simulink model "indy7_dualArm"  (R2024b)
settings: Solver=FixedStepAuto  StartTime=0.0  StopTime=10  FixedStep=0.001  RelTol=1e-3
model workspace (MAT data in the model file):
  joint_friction = [80 80 20 10 10 5]
  lambda_l_list = [0 -1.17357539658 0.993815552956 -2.091 0 0 -0.111945470246 0.0246912114191 0.243747835972 1.20917417944 1.20917417944 -1.20905770917 ... (42 elements, 6x7)]
  lambda_r_list = [0 1.17618914658 0.992300581915 2.091 0 0 -0.111945470246 0.0246912114191 0.243747835972 1.20917417944 1.20917417944 -1.20905770917 ... (42 elements, 6x7)]
  lambda_rl_list = [2.58853268681e-20 -2.25514051877e-16 -0.06 -1.83339582048e-16 -4.06575814682e-20 0 0.0911029490978 -0.02862210596 -0.174516399919 1.20917417944 1.20905770917 -1.20917417944 ... (78 elements, 6x13)]
  q_init_l : Simulink.Parameter (value not decoded)
  q_init_l1 : Simulink.Parameter (value not decoded)
  q_init_l2 : Simulink.Parameter (value not decoded)
  q_init_l3 : Simulink.Parameter (value not decoded)
  q_init_l4 : Simulink.Parameter (value not decoded)
  q_init_l5 : Simulink.Parameter (value not decoded)
  q_init_l6 : Simulink.Parameter (value not decoded)
  q_init_r : Simulink.Parameter (value not decoded)
  q_init_r1 : Simulink.Parameter (value not decoded)
  q_init_r2 : Simulink.Parameter (value not decoded)
  q_init_r3 : Simulink.Parameter (value not decoded)
  q_init_r4 : Simulink.Parameter (value not decoded)
  q_init_r5 : Simulink.Parameter (value not decoded)
  q_init_r6 : Simulink.Parameter (value not decoded)
  robot : robotics.RigidBodyTree (value not decoded)
values from neighbouring files (symbols this model uses):
  lambda_lr_list = [lambda_lr_list,-lambda_rl_list(:,i)]    [getDualArmLambdaList.m]    (also in untitled3.m)
  m = models{k}    [code_generation.m]
  N = length(q)    [FKLocalPOE.m]
symbols that are objects in the model workspace (value not decoded): q_init_l, q_init_l1, q_init_r
undefined symbols (not defined in the file or in its folder): Blist_tcp, DiscIntNeverNeededParam, dt, exp6, M_tcp, q_init, q_max, q_min, qdot_max, qdot_min, SW_a, SW_b0, X, Y, Z
libraries: sm_lib x148, nesl_utility x45, robotmaniplib x9, robotcorelib x5, simulink x4, matrix_library x2
(part 4 of 5)

== system indy7_dualArm/DualArm/Right/r_3 ==
  Inertia : sm_lib/Body Elements/Inertia  InertiaType=Custom  Mass=2.99134127  MassUnits=kg  CenterOfMass=[0, 0, 0]  CenterOfMassUnits=m  MomentsOfInertia=[0.03424593, 0.03406024, 0.00450477]  MomentsOfInertiaUnits=kg*m^2  ProductsOfInertia=[0.00186009, 7.24e-06, 1.49e-06]  ProductsOfInertiaUnits=kg*m^2  GraphicType=None  MarkerShape=Inertia  MarkerSize=20  GraphicVisPropType=SimpleVisualProperties  GraphicDiffuseColor=[0.5 0.5 0.5]  GraphicOpacity=1  GraphicSpecularColor=[0.5 0.5 0.5 1.0]  GraphicAmbientColor=[0.15 0.15 0.15 1.0]  GraphicEmissiveColor=[0.0 0.0 0.0 1.0]  GraphicShininess=75
  InertiaOriginTransform : sm_lib/Frames and Transforms/Rigid Transform  RotationMethod=RotationSequence  FollAlignAxisA=+X  BaseAlignAxisA=+Y  FollAlignAxisB=+Y  BaseAlignAxisB=+Z  RotationStandardAxis=+Z  RotationAngle=0  RotationAngleUnits=deg  RotationArbitraryAxis=[0 0 1]  RotationSequenceAxes=BaseAxes  RotationSequence=XYZ  RotationSequenceAngles=[0, 0, 0]  RotationSequenceAnglesUnits=rad  RotationMatrix=[1 0 0;0 1 0;0 0 1]  Quaternion=[1 0 0 0]  TranslationMethod=Cartesian  TranslationCartesianOffset=[0, 0, 0]  TranslationCartesianOffsetUnits=m  TranslationStandardAxis=+Z  TranslationStandardOffset=0  TranslationStandardOffsetUnits=m  TranslationROffset=0  TranslationROffsetUnits=m  TranslationThetaOffset=0  TranslationThetaOffsetUnits=deg  TranslationZOffset=0  TranslationZOffsetUnits=m
  ReferenceFrame : sm_lib/Frames and Transforms/Reference Frame
  Visual : sm_lib/Body Elements/File Solid  ExtGeomFileName=meshes/visual/Indy7_3.stl  UnitType=Custom  ExtGeomFileUnits=m  StepReaderType=HEX  ExportConvexHullGeometry=off  InertiaType=Custom  BasedOnType=DensityFromFile  Density=1000  DensityUnits=kg/m^3  Mass=0  MassUnits=kg  CenterOfMass=[0, 0, 0]  CenterOfMassUnits=m  MomentsOfInertia=[0, 0, 0]  MomentsOfInertiaUnits=kg*m^2  ProductsOfInertia=[0, 0, 0]  ProductsOfInertiaUnits=kg*m^2  GraphicType=FromGeometry  MarkerShape=Sphere  MarkerSize=10  GraphicVisPropType=SimpleVisualProperties  GraphicDiffuseColor=[1,1,1]  GraphicOpacity=1  GraphicSpecularColor=[0.5 0.5 0.5 1.0]  GraphicAmbientColor=[0.15 0.15 0.15 1.0]  GraphicEmissiveColor=[0.0 0.0 0.0 1.0]  GraphicShininess=75  DoExposeReferenceFrame=on  SerializedFrames=<Frames/>
  VisualOriginTransform : sm_lib/Frames and Transforms/Rigid Transform  RotationMethod=RotationSequence  FollAlignAxisA=+X  BaseAlignAxisA=+Y  FollAlignAxisB=+Y  BaseAlignAxisB=+Z  RotationStandardAxis=+Z  RotationAngle=0  RotationAngleUnits=deg  RotationArbitraryAxis=[0 0 1]  RotationSequenceAxes=BaseAxes  RotationSequence=XYZ  RotationSequenceAngles=[0, 0, 0]  RotationSequenceAnglesUnits=rad  RotationMatrix=[1 0 0;0 1 0;0 0 1]  Quaternion=[1 0 0 0]  TranslationMethod=Cartesian  TranslationCartesianOffset=[0, 0, 0]  TranslationCartesianOffsetUnits=m  TranslationStandardAxis=+Z  TranslationStandardOffset=0  TranslationStandardOffsetUnits=m  TranslationROffset=0  TranslationROffsetUnits=m  TranslationThetaOffset=0  TranslationThetaOffsetUnits=deg  TranslationZOffset=0  TranslationZOffsetUnits=m
  r_joint_2_AxisInvTransform : sm_lib/Frames and Transforms/Rigid Transform  RotationMethod=ArbitraryAxis  FollAlignAxisA=+X  BaseAlignAxisA=+Y  FollAlignAxisB=+Y  BaseAlignAxisB=+Z  RotationStandardAxis=+Z  RotationAngle=0  RotationAngleUnits=rad  RotationArbitraryAxis=[1, 0, 0]  RotationSequenceAxes=FollowerAxes  RotationSequence=XYX  RotationSequenceAngles=[0 0 0]  RotationSequenceAnglesUnits=deg  RotationMatrix=[1 0 0;0 1 0;0 0 1]  Quaternion=[1 0 0 0]  TranslationMethod=Cartesian  TranslationCartesianOffset=[0, 0, 0]  TranslationCartesianOffsetUnits=m  TranslationStandardAxis=+Z  TranslationStandardOffset=0  TranslationStandardOffsetUnits=m  TranslationROffset=0  TranslationROffsetUnits=m  TranslationThetaOffset=0  TranslationThetaOffsetUnits=deg  TranslationZOffset=0  TranslationZOffsetUnits=m
  r_joint_3_AxisTransform : sm_lib/Frames and Transforms/Rigid Transform  RotationMethod=ArbitraryAxis  FollAlignAxisA=+X  BaseAlignAxisA=+Y  FollAlignAxisB=+Y  BaseAlignAxisB=+Z  RotationStandardAxis=+Z  RotationAngle=0  RotationAngleUnits=rad  RotationArbitraryAxis=[1, 0, 0]  RotationSequenceAxes=FollowerAxes  RotationSequence=XYX  RotationSequenceAngles=[0 0 0]  RotationSequenceAnglesUnits=deg  RotationMatrix=[1 0 0;0 1 0;0 0 1]  Quaternion=[1 0 0 0]  TranslationMethod=Cartesian  TranslationCartesianOffset=[0, 0, 0]  TranslationCartesianOffsetUnits=m  TranslationStandardAxis=+Z  TranslationStandardOffset=0  TranslationStandardOffsetUnits=m  TranslationROffset=0  TranslationROffsetUnits=m  TranslationThetaOffset=0  TranslationThetaOffsetUnits=deg  TranslationZOffset=0  TranslationZOffsetUnits=m
  r_joint_3_OriginTransform : sm_lib/Frames and Transforms/Rigid Transform  RotationMethod=RotationSequence  FollAlignAxisA=+X  BaseAlignAxisA=+Y  FollAlignAxisB=+Y  BaseAlignAxisB=+Z  RotationStandardAxis=+Z  RotationAngle=0  RotationAngleUnits=deg  RotationArbitraryAxis=[0 0 1]  RotationSequenceAxes=BaseAxes  RotationSequence=XYZ  RotationSequenceAngles=[-1.5707, 0, 1.5707]  RotationSequenceAnglesUnits=rad  RotationMatrix=[1 0 0;0 1 0;0 0 1]  Quaternion=[1 0 0 0]  TranslationMethod=Cartesian  TranslationCartesianOffset=[-0.267, 0, -0.075]  TranslationCartesianOffsetUnits=m  TranslationStandardAxis=+Z  TranslationStandardOffset=0  TranslationStandardOffsetUnits=m  TranslationROffset=0  TranslationROffsetUnits=m  TranslationThetaOffset=0  TranslationThetaOffsetUnits=deg  TranslationZOffset=0  TranslationZOffsetUnits=m
  F : PMIOPort  Side=Left
  F1 : PMIOPort  Port=2  Side=Right
  connections:
  Inertia/RConn1 -- InertiaOriginTransform/RConn1
  r_joint_2_AxisInvTransform/LConn1 -- r_joint_3_OriginTransform/LConn1 -- InertiaOriginTransform/LConn1 -- ReferenceFrame/RConn1 -- VisualOriginTransform/LConn1
  Visual/RConn1 -- VisualOriginTransform/RConn1
  r_joint_2_AxisInvTransform/RConn1 -- F/RConn1
  r_joint_3_AxisTransform/RConn1 -- F1/RConn1
  r_joint_3_AxisTransform/LConn1 -- r_joint_3_OriginTransform/RConn1

== system indy7_dualArm/DualArm/Right/r_4 ==
  Inertia : sm_lib/Body Elements/Inertia  InertiaType=Custom  Mass=2.12317035  MassUnits=kg  CenterOfMass=[0, 0, 0]  CenterOfMassUnits=m  MomentsOfInertia=[0.00670405, 0.00279246, 0.00619341]  MomentsOfInertiaUnits=kg*m^2  ProductsOfInertia=[-0.00127967, 1.5e-06, 3.75e-06]  ProductsOfInertiaUnits=kg*m^2  GraphicType=None  MarkerShape=Inertia  MarkerSize=20  GraphicVisPropType=SimpleVisualProperties  GraphicDiffuseColor=[0.5 0.5 0.5]  GraphicOpacity=1  GraphicSpecularColor=[0.5 0.5 0.5 1.0]  GraphicAmbientColor=[0.15 0.15 0.15 1.0]  GraphicEmissiveColor=[0.0 0.0 0.0 1.0]  GraphicShininess=75
  InertiaOriginTransform : sm_lib/Frames and Transforms/Rigid Transform  RotationMethod=RotationSequence  FollAlignAxisA=+X  BaseAlignAxisA=+Y  FollAlignAxisB=+Y  BaseAlignAxisB=+Z  RotationStandardAxis=+Z  RotationAngle=0  RotationAngleUnits=deg  RotationArbitraryAxis=[0 0 1]  RotationSequenceAxes=BaseAxes  RotationSequence=XYZ  RotationSequenceAngles=[0, 0, 0]  RotationSequenceAnglesUnits=rad  RotationMatrix=[1 0 0;0 1 0;0 0 1]  Quaternion=[1 0 0 0]  TranslationMethod=Cartesian  TranslationCartesianOffset=[0, 0, 0]  TranslationCartesianOffsetUnits=m  TranslationStandardAxis=+Z  TranslationStandardOffset=0  TranslationStandardOffsetUnits=m  TranslationROffset=0  TranslationROffsetUnits=m  TranslationThetaOffset=0  TranslationThetaOffsetUnits=deg  TranslationZOffset=0  TranslationZOffsetUnits=m
  ReferenceFrame : sm_lib/Frames and Transforms/Reference Frame
  Visual : sm_lib/Body Elements/File Solid  ExtGeomFileName=meshes/visual/Indy7_4.stl  UnitType=Custom  ExtGeomFileUnits=m  StepReaderType=HEX  ExportConvexHullGeometry=off  InertiaType=Custom  BasedOnType=DensityFromFile  Density=1000  DensityUnits=kg/m^3  Mass=0  MassUnits=kg  CenterOfMass=[0, 0, 0]  CenterOfMassUnits=m  MomentsOfInertia=[0, 0, 0]  MomentsOfInertiaUnits=kg*m^2  ProductsOfInertia=[0, 0, 0]  ProductsOfInertiaUnits=kg*m^2  GraphicType=FromGeometry  MarkerShape=Sphere  MarkerSize=10  GraphicVisPropType=SimpleVisualProperties  GraphicDiffuseColor=[1,1,1]  GraphicOpacity=1  GraphicSpecularColor=[0.5 0.5 0.5 1.0]  GraphicAmbientColor=[0.15 0.15 0.15 1.0]  GraphicEmissiveColor=[0.0 0.0 0.0 1.0]  GraphicShininess=75  DoExposeReferenceFrame=on  SerializedFrames=<Frames/>
  VisualOriginTransform : sm_lib/Frames and Transforms/Rigid Transform  RotationMethod=RotationSequence  FollAlignAxisA=+X  BaseAlignAxisA=+Y  FollAlignAxisB=+Y  BaseAlignAxisB=+Z  RotationStandardAxis=+Z  RotationAngle=0  RotationAngleUnits=deg  RotationArbitraryAxis=[0 0 1]  RotationSequenceAxes=BaseAxes  RotationSequence=XYZ  RotationSequenceAngles=[0, 0, 0]  RotationSequenceAnglesUnits=rad  RotationMatrix=[1 0 0;0 1 0;0 0 1]  Quaternion=[1 0 0 0]  TranslationMethod=Cartesian  TranslationCartesianOffset=[0, 0, 0]  TranslationCartesianOffsetUnits=m  TranslationStandardAxis=+Z  TranslationStandardOffset=0  TranslationStandardOffsetUnits=m  TranslationROffset=0  TranslationROffsetUnits=m  TranslationThetaOffset=0  TranslationThetaOffsetUnits=deg  TranslationZOffset=0  TranslationZOffsetUnits=m
  r_joint_3_AxisInvTransform : sm_lib/Frames and Transforms/Rigid Transform  RotationMethod=ArbitraryAxis  FollAlignAxisA=+X  BaseAlignAxisA=+Y  FollAlignAxisB=+Y  BaseAlignAxisB=+Z  RotationStandardAxis=+Z  RotationAngle=0  RotationAngleUnits=rad  RotationArbitraryAxis=[1, 0, 0]  RotationSequenceAxes=FollowerAxes  RotationSequence=XYX  RotationSequenceAngles=[0 0 0]  RotationSequenceAnglesUnits=deg  RotationMatrix=[1 0 0;0 1 0;0 0 1]  Quaternion=[1 0 0 0]  TranslationMethod=Cartesian  TranslationCartesianOffset=[0, 0, 0]  TranslationCartesianOffsetUnits=m  TranslationStandardAxis=+Z  TranslationStandardOffset=0  TranslationStandardOffsetUnits=m  TranslationROffset=0  TranslationROffsetUnits=m  TranslationThetaOffset=0  TranslationThetaOffsetUnits=deg  TranslationZOffset=0  TranslationZOffsetUnits=m
  r_joint_4_AxisTransform : sm_lib/Frames and Transforms/Rigid Transform  RotationMethod=ArbitraryAxis  FollAlignAxisA=+X  BaseAlignAxisA=+Y  FollAlignAxisB=+Y  BaseAlignAxisB=+Z  RotationStandardAxis=+Z  RotationAngle=0  RotationAngleUnits=rad  RotationArbitraryAxis=[1, 0, 0]  RotationSequenceAxes=FollowerAxes  RotationSequence=XYX  RotationSequenceAngles=[0 0 0]  RotationSequenceAnglesUnits=deg  RotationMatrix=[1 0 0;0 1 0;0 0 1]  Quaternion=[1 0 0 0]  TranslationMethod=Cartesian  TranslationCartesianOffset=[0, 0, 0]  TranslationCartesianOffsetUnits=m  TranslationStandardAxis=+Z  TranslationStandardOffset=0  TranslationStandardOffsetUnits=m  TranslationROffset=0  TranslationROffsetUnits=m  TranslationThetaOffset=0  TranslationThetaOffsetUnits=deg  TranslationZOffset=0  TranslationZOffsetUnits=m
  r_joint_4_OriginTransform : sm_lib/Frames and Transforms/Rigid Transform  RotationMethod=RotationSequence  FollAlignAxisA=+X  BaseAlignAxisA=+Y  FollAlignAxisB=+Y  BaseAlignAxisB=+Z  RotationStandardAxis=+Z  RotationAngle=0  RotationAngleUnits=deg  RotationArbitraryAxis=[0 0 1]  RotationSequenceAxes=BaseAxes  RotationSequence=XYZ  RotationSequenceAngles=[1.5707, 1.5707, 0]  RotationSequenceAnglesUnits=rad  RotationMatrix=[1 0 0;0 1 0;0 0 1]  Quaternion=[1 0 0 0]  TranslationMethod=Cartesian  TranslationCartesianOffset=[0, -0.114, 0.083]  TranslationCartesianOffsetUnits=m  TranslationStandardAxis=+Z  TranslationStandardOffset=0  TranslationStandardOffsetUnits=m  TranslationROffset=0  TranslationROffsetUnits=m  TranslationThetaOffset=0  TranslationThetaOffsetUnits=deg  TranslationZOffset=0  TranslationZOffsetUnits=m
  F : PMIOPort  Side=Left
  F1 : PMIOPort  Port=2  Side=Right
  connections:
  Inertia/RConn1 -- InertiaOriginTransform/RConn1
  r_joint_3_AxisInvTransform/LConn1 -- r_joint_4_OriginTransform/LConn1 -- InertiaOriginTransform/LConn1 -- ReferenceFrame/RConn1 -- VisualOriginTransform/LConn1
  Visual/RConn1 -- VisualOriginTransform/RConn1
  r_joint_3_AxisInvTransform/RConn1 -- F/RConn1
  r_joint_4_AxisTransform/RConn1 -- F1/RConn1
  r_joint_4_AxisTransform/LConn1 -- r_joint_4_OriginTransform/RConn1

== system indy7_dualArm/DualArm/Right/r_5 ==
  Inertia : sm_lib/Body Elements/Inertia  InertiaType=Custom  Mass=2.28865091  MassUnits=kg  CenterOfMass=[0, 0, 0]  CenterOfMassUnits=m  MomentsOfInertia=[0.00994891, 0.00978189, 0.00271492]  MomentsOfInertiaUnits=kg*m^2  ProductsOfInertia=[-0.00093546, 3.21e-06, 1.4e-07]  ProductsOfInertiaUnits=kg*m^2  GraphicType=None  MarkerShape=Inertia  MarkerSize=20  GraphicVisPropType=SimpleVisualProperties  GraphicDiffuseColor=[0.5 0.5 0.5]  GraphicOpacity=1  GraphicSpecularColor=[0.5 0.5 0.5 1.0]  GraphicAmbientColor=[0.15 0.15 0.15 1.0]  GraphicEmissiveColor=[0.0 0.0 0.0 1.0]  GraphicShininess=75
  InertiaOriginTransform : sm_lib/Frames and Transforms/Rigid Transform  RotationMethod=RotationSequence  FollAlignAxisA=+X  BaseAlignAxisA=+Y  FollAlignAxisB=+Y  BaseAlignAxisB=+Z  RotationStandardAxis=+Z  RotationAngle=0  RotationAngleUnits=deg  RotationArbitraryAxis=[0 0 1]  RotationSequenceAxes=BaseAxes  RotationSequence=XYZ  RotationSequenceAngles=[0, 0, 0]  RotationSequenceAnglesUnits=rad  RotationMatrix=[1 0 0;0 1 0;0 0 1]  Quaternion=[1 0 0 0]  TranslationMethod=Cartesian  TranslationCartesianOffset=[0, 0, 0]  TranslationCartesianOffsetUnits=m  TranslationStandardAxis=+Z  TranslationStandardOffset=0  TranslationStandardOffsetUnits=m  TranslationROffset=0  TranslationROffsetUnits=m  TranslationThetaOffset=0  TranslationThetaOffsetUnits=deg  TranslationZOffset=0  TranslationZOffsetUnits=m
  ReferenceFrame : sm_lib/Frames and Transforms/Reference Frame
  Visual : sm_lib/Body Elements/File Solid  ExtGeomFileName=meshes/visual/Indy7_5.stl  UnitType=Custom  ExtGeomFileUnits=m  StepReaderType=HEX  ExportConvexHullGeometry=off  InertiaType=Custom  BasedOnType=DensityFromFile  Density=1000  DensityUnits=kg/m^3  Mass=0  MassUnits=kg  CenterOfMass=[0, 0, 0]  CenterOfMassUnits=m  MomentsOfInertia=[0, 0, 0]  MomentsOfInertiaUnits=kg*m^2  ProductsOfInertia=[0, 0, 0]  ProductsOfInertiaUnits=kg*m^2  GraphicType=FromGeometry  MarkerShape=Sphere  MarkerSize=10  GraphicVisPropType=SimpleVisualProperties  GraphicDiffuseColor=[1,1,1]  GraphicOpacity=1  GraphicSpecularColor=[0.5 0.5 0.5 1.0]  GraphicAmbientColor=[0.15 0.15 0.15 1.0]  GraphicEmissiveColor=[0.0 0.0 0.0 1.0]  GraphicShininess=75  DoExposeReferenceFrame=on  SerializedFrames=<Frames/>
  VisualOriginTransform : sm_lib/Frames and Transforms/Rigid Transform  RotationMethod=RotationSequence  FollAlignAxisA=+X  BaseAlignAxisA=+Y  FollAlignAxisB=+Y  BaseAlignAxisB=+Z  RotationStandardAxis=+Z  RotationAngle=0  RotationAngleUnits=deg  RotationArbitraryAxis=[0 0 1]  RotationSequenceAxes=BaseAxes  RotationSequence=XYZ  RotationSequenceAngles=[0, 0, 0]  RotationSequenceAnglesUnits=rad  RotationMatrix=[1 0 0;0 1 0;0 0 1]  Quaternion=[1 0 0 0]  TranslationMethod=Cartesian  TranslationCartesianOffset=[0, 0, 0]  TranslationCartesianOffsetUnits=m  TranslationStandardAxis=+Z  TranslationStandardOffset=0  TranslationStandardOffsetUnits=m  TranslationROffset=0  TranslationROffsetUnits=m  TranslationThetaOffset=0  TranslationThetaOffsetUnits=deg  TranslationZOffset=0  TranslationZOffsetUnits=m
  r_joint_4_AxisInvTransform : sm_lib/Frames and Transforms/Rigid Transform  RotationMethod=ArbitraryAxis  FollAlignAxisA=+X  BaseAlignAxisA=+Y  FollAlignAxisB=+Y  BaseAlignAxisB=+Z  RotationStandardAxis=+Z  RotationAngle=0  RotationAngleUnits=rad  RotationArbitraryAxis=[1, 0, 0]  RotationSequenceAxes=FollowerAxes  RotationSequence=XYX  RotationSequenceAngles=[0 0 0]  RotationSequenceAnglesUnits=deg  RotationMatrix=[1 0 0;0 1 0;0 0 1]  Quaternion=[1 0 0 0]  TranslationMethod=Cartesian  TranslationCartesianOffset=[0, 0, 0]  TranslationCartesianOffsetUnits=m  TranslationStandardAxis=+Z  TranslationStandardOffset=0  TranslationStandardOffsetUnits=m  TranslationROffset=0  TranslationROffsetUnits=m  TranslationThetaOffset=0  TranslationThetaOffsetUnits=deg  TranslationZOffset=0  TranslationZOffsetUnits=m
  r_joint_5_AxisTransform : sm_lib/Frames and Transforms/Rigid Transform  RotationMethod=ArbitraryAxis  FollAlignAxisA=+X  BaseAlignAxisA=+Y  FollAlignAxisB=+Y  BaseAlignAxisB=+Z  RotationStandardAxis=+Z  RotationAngle=0  RotationAngleUnits=rad  RotationArbitraryAxis=[1, 0, 0]  RotationSequenceAxes=FollowerAxes  RotationSequence=XYX  RotationSequenceAngles=[0 0 0]  RotationSequenceAnglesUnits=deg  RotationMatrix=[1 0 0;0 1 0;0 0 1]  Quaternion=[1 0 0 0]  TranslationMethod=Cartesian  TranslationCartesianOffset=[0, 0, 0]  TranslationCartesianOffsetUnits=m  TranslationStandardAxis=+Z  TranslationStandardOffset=0  TranslationStandardOffsetUnits=m  TranslationROffset=0  TranslationROffsetUnits=m  TranslationThetaOffset=0  TranslationThetaOffsetUnits=deg  TranslationZOffset=0  TranslationZOffsetUnits=m
  r_joint_5_OriginTransform : sm_lib/Frames and Transforms/Rigid Transform  RotationMethod=RotationSequence  FollAlignAxisA=+X  BaseAlignAxisA=+Y  FollAlignAxisB=+Y  BaseAlignAxisB=+Z  RotationStandardAxis=+Z  RotationAngle=0  RotationAngleUnits=deg  RotationArbitraryAxis=[0 0 1]  RotationSequenceAxes=BaseAxes  RotationSequence=XYZ  RotationSequenceAngles=[-1.5707, 0, 1.5707]  RotationSequenceAnglesUnits=rad  RotationMatrix=[1 0 0;0 1 0;0 0 1]  Quaternion=[1 0 0 0]  TranslationMethod=Cartesian  TranslationCartesianOffset=[-0.168, 0, 0.06900000000000001]  TranslationCartesianOffsetUnits=m  TranslationStandardAxis=+Z  TranslationStandardOffset=0  TranslationStandardOffsetUnits=m  TranslationROffset=0  TranslationROffsetUnits=m  TranslationThetaOffset=0  TranslationThetaOffsetUnits=deg  TranslationZOffset=0  TranslationZOffsetUnits=m
  F : PMIOPort  Side=Left
  F1 : PMIOPort  Port=2  Side=Right
  connections:
  Inertia/RConn1 -- InertiaOriginTransform/RConn1
  r_joint_4_AxisInvTransform/LConn1 -- r_joint_5_OriginTransform/LConn1 -- InertiaOriginTransform/LConn1 -- ReferenceFrame/RConn1 -- VisualOriginTransform/LConn1
  Visual/RConn1 -- VisualOriginTransform/RConn1
  r_joint_4_AxisInvTransform/RConn1 -- F/RConn1
  r_joint_5_AxisTransform/RConn1 -- F1/RConn1
  r_joint_5_AxisTransform/LConn1 -- r_joint_5_OriginTransform/RConn1

== system indy7_dualArm/DualArm/Right/r_6 ==
  Inertia : sm_lib/Body Elements/Inertia  InertiaType=Custom  Mass=0.40083918  MassUnits=kg  CenterOfMass=[0, 0, 0]  CenterOfMassUnits=m  MomentsOfInertia=[0.00043534, 0.00044549, 0.00059634]  MomentsOfInertiaUnits=kg*m^2  ProductsOfInertia=[5.1e-07, -2e-08, 1.3e-07]  ProductsOfInertiaUnits=kg*m^2  GraphicType=None  MarkerShape=Inertia  MarkerSize=20  GraphicVisPropType=SimpleVisualProperties  GraphicDiffuseColor=[0.5 0.5 0.5]  GraphicOpacity=1  GraphicSpecularColor=[0.5 0.5 0.5 1.0]  GraphicAmbientColor=[0.15 0.15 0.15 1.0]  GraphicEmissiveColor=[0.0 0.0 0.0 1.0]  GraphicShininess=75
  InertiaOriginTransform : sm_lib/Frames and Transforms/Rigid Transform  RotationMethod=RotationSequence  FollAlignAxisA=+X  BaseAlignAxisA=+Y  FollAlignAxisB=+Y  BaseAlignAxisB=+Z  RotationStandardAxis=+Z  RotationAngle=0  RotationAngleUnits=deg  RotationArbitraryAxis=[0 0 1]  RotationSequenceAxes=BaseAxes  RotationSequence=XYZ  RotationSequenceAngles=[0, 0, 0]  RotationSequenceAnglesUnits=rad  RotationMatrix=[1 0 0;0 1 0;0 0 1]  Quaternion=[1 0 0 0]  TranslationMethod=Cartesian  TranslationCartesianOffset=[0, 0, 0]  TranslationCartesianOffsetUnits=m  TranslationStandardAxis=+Z  TranslationStandardOffset=0  TranslationStandardOffsetUnits=m  TranslationROffset=0  TranslationROffsetUnits=m  TranslationThetaOffset=0  TranslationThetaOffsetUnits=deg  TranslationZOffset=0  TranslationZOffsetUnits=m
  ReferenceFrame : sm_lib/Frames and Transforms/Reference Frame
  Visual : sm_lib/Body Elements/File Solid  ExtGeomFileName=meshes/visual/Indy7_6.stl  UnitType=Custom  ExtGeomFileUnits=m  StepReaderType=HEX  ExportConvexHullGeometry=off  InertiaType=Custom  BasedOnType=DensityFromFile  Density=1000  DensityUnits=kg/m^3  Mass=0  MassUnits=kg  CenterOfMass=[0, 0, 0]  CenterOfMassUnits=m  MomentsOfInertia=[0, 0, 0]  MomentsOfInertiaUnits=kg*m^2  ProductsOfInertia=[0, 0, 0]  ProductsOfInertiaUnits=kg*m^2  GraphicType=FromGeometry  MarkerShape=Sphere  MarkerSize=10  GraphicVisPropType=SimpleVisualProperties  GraphicDiffuseColor=[1,1,1]  GraphicOpacity=1  GraphicSpecularColor=[0.5 0.5 0.5 1.0]  GraphicAmbientColor=[0.15 0.15 0.15 1.0]  GraphicEmissiveColor=[0.0 0.0 0.0 1.0]  GraphicShininess=75  DoExposeReferenceFrame=on  SerializedFrames=<Frames/>
  VisualOriginTransform : sm_lib/Frames and Transforms/Rigid Transform  RotationMethod=RotationSequence  FollAlignAxisA=+X  BaseAlignAxisA=+Y  FollAlignAxisB=+Y  BaseAlignAxisB=+Z  RotationStandardAxis=+Z  RotationAngle=0  RotationAngleUnits=deg  RotationArbitraryAxis=[0 0 1]  RotationSequenceAxes=BaseAxes  RotationSequence=XYZ  RotationSequenceAngles=[0, 0, 0]  RotationSequenceAnglesUnits=rad  RotationMatrix=[1 0 0;0 1 0;0 0 1]  Quaternion=[1 0 0 0]  TranslationMethod=Cartesian  TranslationCartesianOffset=[0, 0, 0]  TranslationCartesianOffsetUnits=m  TranslationStandardAxis=+Z  TranslationStandardOffset=0  TranslationStandardOffsetUnits=m  TranslationROffset=0  TranslationROffsetUnits=m  TranslationThetaOffset=0  TranslationThetaOffsetUnits=deg  TranslationZOffset=0  TranslationZOffsetUnits=m
  r_joint_5_AxisInvTransform : sm_lib/Frames and Transforms/Rigid Transform  RotationMethod=ArbitraryAxis  FollAlignAxisA=+X  BaseAlignAxisA=+Y  FollAlignAxisB=+Y  BaseAlignAxisB=+Z  RotationStandardAxis=+Z  RotationAngle=0  RotationAngleUnits=rad  RotationArbitraryAxis=[1, 0, 0]  RotationSequenceAxes=FollowerAxes  RotationSequence=XYX  RotationSequenceAngles=[0 0 0]  RotationSequenceAnglesUnits=deg  RotationMatrix=[1 0 0;0 1 0;0 0 1]  Quaternion=[1 0 0 0]  TranslationMethod=Cartesian  TranslationCartesianOffset=[0, 0, 0]  TranslationCartesianOffsetUnits=m  TranslationStandardAxis=+Z  TranslationStandardOffset=0  TranslationStandardOffsetUnits=m  TranslationROffset=0  TranslationROffsetUnits=m  TranslationThetaOffset=0  TranslationThetaOffsetUnits=deg  TranslationZOffset=0  TranslationZOffsetUnits=m
  r_joint_tcp_OriginTransform : sm_lib/Frames and Transforms/Rigid Transform  RotationMethod=RotationSequence  FollAlignAxisA=+X  BaseAlignAxisA=+Y  FollAlignAxisB=+Y  BaseAlignAxisB=+Z  RotationStandardAxis=+Z  RotationAngle=0  RotationAngleUnits=deg  RotationArbitraryAxis=[0 0 1]  RotationSequenceAxes=BaseAxes  RotationSequence=XYZ  RotationSequenceAngles=[0, 0, 0]  RotationSequenceAnglesUnits=rad  RotationMatrix=[1 0 0;0 1 0;0 0 1]  Quaternion=[1 0 0 0]  TranslationMethod=Cartesian  TranslationCartesianOffset=[0, 0, 0.06]  TranslationCartesianOffsetUnits=m  TranslationStandardAxis=+Z  TranslationStandardOffset=0  TranslationStandardOffsetUnits=m  TranslationROffset=0  TranslationROffsetUnits=m  TranslationThetaOffset=0  TranslationThetaOffsetUnits=deg  TranslationZOffset=0  TranslationZOffsetUnits=m
  F : PMIOPort  Side=Left
  F1 : PMIOPort  Port=2  Side=Right
  connections:
  Inertia/RConn1 -- InertiaOriginTransform/RConn1
  r_joint_5_AxisInvTransform/LConn1 -- r_joint_tcp_OriginTransform/LConn1 -- InertiaOriginTransform/LConn1 -- ReferenceFrame/RConn1 -- VisualOriginTransform/LConn1
  Visual/RConn1 -- VisualOriginTransform/RConn1
  r_joint_5_AxisInvTransform/RConn1 -- F/RConn1
  r_joint_tcp_OriginTransform/RConn1 -- F1/RConn1

== system indy7_dualArm/DualArm/Right/r_tcp ==
  Inertia : sm_lib/Body Elements/Inertia  InertiaType=Custom  Mass=0  MassUnits=kg  CenterOfMass=[0, 0, 0]  CenterOfMassUnits=m  MomentsOfInertia=[0, 0, 0]  MomentsOfInertiaUnits=kg*m^2  ProductsOfInertia=[0, 0, 0]  ProductsOfInertiaUnits=kg*m^2  GraphicType=None  MarkerShape=Inertia  MarkerSize=20  GraphicVisPropType=SimpleVisualProperties  GraphicDiffuseColor=[0.5 0.5 0.5]  GraphicOpacity=1  GraphicSpecularColor=[0.5 0.5 0.5 1.0]  GraphicAmbientColor=[0.15 0.15 0.15 1.0]  GraphicEmissiveColor=[0.0 0.0 0.0 1.0]  GraphicShininess=75
  InertiaOriginTransform : sm_lib/Frames and Transforms/Rigid Transform  RotationMethod=RotationSequence  FollAlignAxisA=+X  BaseAlignAxisA=+Y  FollAlignAxisB=+Y  BaseAlignAxisB=+Z  RotationStandardAxis=+Z  RotationAngle=0  RotationAngleUnits=deg  RotationArbitraryAxis=[0 0 1]  RotationSequenceAxes=BaseAxes  RotationSequence=XYZ  RotationSequenceAngles=[0, 0, 0]  RotationSequenceAnglesUnits=rad  RotationMatrix=[1 0 0;0 1 0;0 0 1]  Quaternion=[1 0 0 0]  TranslationMethod=Cartesian  TranslationCartesianOffset=[0, 0, 0]  TranslationCartesianOffsetUnits=m  TranslationStandardAxis=+Z  TranslationStandardOffset=0  TranslationStandardOffsetUnits=m  TranslationROffset=0  TranslationROffsetUnits=m  TranslationThetaOffset=0  TranslationThetaOffsetUnits=deg  TranslationZOffset=0  TranslationZOffsetUnits=m
  ReferenceFrame : sm_lib/Frames and Transforms/Reference Frame
  VisualOriginTransform : sm_lib/Frames and Transforms/Rigid Transform  RotationMethod=RotationSequence  FollAlignAxisA=+X  BaseAlignAxisA=+Y  FollAlignAxisB=+Y  BaseAlignAxisB=+Z  RotationStandardAxis=+Z  RotationAngle=0  RotationAngleUnits=deg  RotationArbitraryAxis=[0 0 1]  RotationSequenceAxes=BaseAxes  RotationSequence=XYZ  RotationSequenceAngles=[1.570796, 0, 0]  RotationSequenceAnglesUnits=rad  RotationMatrix=[1 0 0;0 1 0;0 0 1]  Quaternion=[1 0 0 0]  TranslationMethod=Cartesian  TranslationCartesianOffset=[0, 0, 0]  TranslationCartesianOffsetUnits=m  TranslationStandardAxis=+Z  TranslationStandardOffset=0  TranslationStandardOffsetUnits=m  TranslationROffset=0  TranslationROffsetUnits=m  TranslationThetaOffset=0  TranslationThetaOffsetUnits=deg  TranslationZOffset=0  TranslationZOffsetUnits=m
  F : PMIOPort  Side=Left
  Connection Port : PMIOPort  Port=2  Side=Left
  connections:
  Inertia/RConn1 -- InertiaOriginTransform/RConn1
  ReferenceFrame/RConn1 -- F/RConn1 -- InertiaOriginTransform/LConn1 -- VisualOriginTransform/LConn1
  Connection Port/RConn1 -- VisualOriginTransform/RConn1

== system indy7_dualArm/DualArm/Subsystem/body1 ==
  Inertia : sm_lib/Body Elements/Inertia  InertiaType=Custom  Mass=1.59306955  MassUnits=kg  CenterOfMass=[0, 0, 0]  CenterOfMassUnits=m  MomentsOfInertia=[0.00572623, 0.00558959, 0.00966674]  MomentsOfInertiaUnits=kg*m^2  ProductsOfInertia=[-1.4e-07, -0.0001138, 2.51e-06]  ProductsOfInertiaUnits=kg*m^2  GraphicType=None  MarkerShape=Inertia  MarkerSize=20  GraphicVisPropType=SimpleVisualProperties  GraphicDiffuseColor=[0.5 0.5 0.5]  GraphicOpacity=1  GraphicSpecularColor=[0.5 0.5 0.5 1.0]  GraphicAmbientColor=[0.15 0.15 0.15 1.0]  GraphicEmissiveColor=[0.0 0.0 0.0 1.0]  GraphicShininess=75
  InertiaOriginTransform : sm_lib/Frames and Transforms/Rigid Transform  RotationMethod=RotationSequence  FollAlignAxisA=+X  BaseAlignAxisA=+Y  FollAlignAxisB=+Y  BaseAlignAxisB=+Z  RotationStandardAxis=+Z  RotationAngle=0  RotationAngleUnits=deg  RotationArbitraryAxis=[0 0 1]  RotationSequenceAxes=BaseAxes  RotationSequence=XYZ  RotationSequenceAngles=[0, 0, 0]  RotationSequenceAnglesUnits=rad  RotationMatrix=[1 0 0;0 1 0;0 0 1]  Quaternion=[1 0 0 0]  TranslationMethod=Cartesian  TranslationCartesianOffset=[0, 0, 0]  TranslationCartesianOffsetUnits=m  TranslationStandardAxis=+Z  TranslationStandardOffset=0  TranslationStandardOffsetUnits=m  TranslationROffset=0  TranslationROffsetUnits=m  TranslationThetaOffset=0  TranslationThetaOffsetUnits=deg  TranslationZOffset=0  TranslationZOffsetUnits=m
  ReferenceFrame : sm_lib/Frames and Transforms/Reference Frame
  Visual : sm_lib/Body Elements/File Solid  ExtGeomFileName=meshes/dual_arm_body.stl  UnitType=Custom  ExtGeomFileUnits=m  StepReaderType=HEX  ExportConvexHullGeometry=off  InertiaType=Custom  BasedOnType=DensityFromFile  Density=1000  DensityUnits=kg/m^3  Mass=0  MassUnits=kg  CenterOfMass=[0, 0, 0]  CenterOfMassUnits=m  MomentsOfInertia=[0, 0, 0]  MomentsOfInertiaUnits=kg*m^2  ProductsOfInertia=[0, 0, 0]  ProductsOfInertiaUnits=kg*m^2  GraphicType=FromGeometry  MarkerShape=Sphere  MarkerSize=10  GraphicVisPropType=SimpleVisualProperties  GraphicDiffuseColor=[0.5, 0.5, 0.5]  GraphicOpacity=1  GraphicSpecularColor=[0.5 0.5 0.5 1.0]  GraphicAmbientColor=[0.15 0.15 0.15 1.0]  GraphicEmissiveColor=[0.0 0.0 0.0 1.0]  GraphicShininess=75  DoExposeReferenceFrame=on  SerializedFrames=<Frames/>
  VisualOriginTransform : sm_lib/Frames and Transforms/Rigid Transform  RotationMethod=RotationSequence  FollAlignAxisA=+X  BaseAlignAxisA=+Y  FollAlignAxisB=+Y  BaseAlignAxisB=+Z  RotationStandardAxis=+Z  RotationAngle=0  RotationAngleUnits=deg  RotationArbitraryAxis=[0 0 1]  RotationSequenceAxes=BaseAxes  RotationSequence=XYZ  RotationSequenceAngles=[0, 0, 0]  RotationSequenceAnglesUnits=rad  RotationMatrix=[1 0 0;0 1 0;0 0 1]  Quaternion=[1 0 0 0]  TranslationMethod=Cartesian  TranslationCartesianOffset=[0, 0, 0]  TranslationCartesianOffsetUnits=m  TranslationStandardAxis=+Z  TranslationStandardOffset=0  TranslationStandardOffsetUnits=m  TranslationROffset=0  TranslationROffsetUnits=m  TranslationThetaOffset=0  TranslationThetaOffsetUnits=deg  TranslationZOffset=0  TranslationZOffsetUnits=m
  l_body_fixed_OriginTransform : sm_lib/Frames and Transforms/Rigid Transform  RotationMethod=RotationSequence  FollAlignAxisA=+X  BaseAlignAxisA=+Y  FollAlignAxisB=+Y  BaseAlignAxisB=+Z  RotationStandardAxis=+Z  RotationAngle=0  RotationAngleUnits=deg  RotationArbitraryAxis=[0 0 1]  RotationSequenceAxes=BaseAxes  RotationSequence=XYZ  RotationSequenceAngles=[-2.091, 0, 0]  RotationSequenceAnglesUnits=rad  RotationMatrix=[1 0 0;0 1 0;0 0 1]  Quaternion=[1 0 0 0]  TranslationMethod=Cartesian  TranslationCartesianOffset=[0, 0.1551, 1.2924]  TranslationCartesianOffsetUnits=m  TranslationStandardAxis=+Z  TranslationStandardOffset=0  TranslationStandardOffsetUnits=m  TranslationROffset=0  TranslationROffsetUnits=m  TranslationThetaOffset=0  TranslationThetaOffsetUnits=deg  TranslationZOffset=0  TranslationZOffsetUnits=m
  r_body_fixed_OriginTransform : sm_lib/Frames and Transforms/Rigid Transform  RotationMethod=RotationSequence  FollAlignAxisA=+X  BaseAlignAxisA=+Y  FollAlignAxisB=+Y  BaseAlignAxisB=+Z  RotationStandardAxis=+Z  RotationAngle=0  RotationAngleUnits=deg  RotationArbitraryAxis=[0 0 1]  RotationSequenceAxes=BaseAxes  RotationSequence=XYZ  RotationSequenceAngles=[2.091, 0, 0]  RotationSequenceAnglesUnits=rad  RotationMatrix=[1 0 0;0 1 0;0 0 1]  Quaternion=[1 0 0 0]  TranslationMethod=Cartesian  TranslationCartesianOffset=[0, -0.1551, 1.2924]  TranslationCartesianOffsetUnits=m  TranslationStandardAxis=+Z  TranslationStandardOffset=0  TranslationStandardOffsetUnits=m  TranslationROffset=0  TranslationROffsetUnits=m  TranslationThetaOffset=0  TranslationThetaOffsetUnits=deg  TranslationZOffset=0  TranslationZOffsetUnits=m
  F : PMIOPort  Side=Left
  F2 : PMIOPort  Port=2  Side=Right
  F1 : PMIOPort  Port=3  Side=Right
  connections:
  Inertia/RConn1 -- InertiaOriginTransform/RConn1
  InertiaOriginTransform/LConn1 -- ReferenceFrame/RConn1 -- F/RConn1 -- l_body_fixed_OriginTransform/LConn1 -- r_body_fixed_OriginTransform/LConn1 -- VisualOriginTransform/LConn1
  Visual/RConn1 -- VisualOriginTransform/RConn1
  l_body_fixed_OriginTransform/RConn1 -- F1/RConn1
  r_body_fixed_OriginTransform/RConn1 -- F2/RConn1

== matlab function indy7_dualArm/Kinematics/MATLAB Function8 ==
  data: Jdot output; J output; lambda_list input; T output; q input; q_dot input
function [Jdot,J,T]=FKJacobian(lambda_list,q,q_dot)
    Ti = eye(4);
    [m,n]=size(lambda_list);
    lamda_z = [0,0,0,0,0,1]';
    ez = [0,0,1]';
    N = length(q);
    J = zeros(6,N);
    Jdot=zeros(6,N);
  
    Ti = exp6(lambda_list(:,end));
    [Ri,pi] = TransToRp(Ti);
    J(:,end)=[Ri'*VecToso3(ez)*pi;Ri'*ez];
    for i =N:-1:1
        Ti = exp6(lambda_list(:,i))*exp6(lamda_z*q(i))*Ti;
 
        [Ri,pi] = TransToRp(Ti);
        if i>1
            J(:,i-1)=[Ri'*VecToso3(ez)*pi;Ri'*ez];
        end

    end
    for i=1:1:N
        Ji = J(:,i);
        dJidt = zeros(6,1);
        for j=1:1:N
            Jj = J(:,j);
            aJiaqj = zeros(6,1);
            if(i<j) 
                aJiaqj = ad(Ji)*Jj;
            end
            dJidt = dJidt+aJiaqj*q_dot(j);
        end
        Jdot(:,i) = dJidt;
    end
    T = Ti;
end

== matlab function indy7_dualArm/Subsystem/GetT,V,Vdot ==
  data: p_t input; T_t output; pdot_t input; pddot_t input; R_t input; omega_t input; omegadot_t input; V_t output; Vdot_t output
function [T_t,V_t,Vdot_t] = getTVVdot(p_t,pdot_t,pddot_t,R_t,omega_t,omegadot_t)

T_t = RpToTrans(R_t,p_t);
V_t = [R_t'*pdot_t;omega_t];
Rdot_t = (R_t*VecToso3(omega_t))';
Vdot_t = [Rdot_t'*pdot_t+R_t'*pddot_t;omegadot_t];

== matlab function indy7_dualArm/Subsystem/MATLAB Function ==
  data: Rstart input; xi_start output; Rend input; xi_end output
function [xi_start,xi_end] = fcn(Rstart,Rend)

xi_start = zeros(3,1);
xi_end = zeros(3,1);

xi_end = so3ToVec(MatrixLog3((Rstart)'*Rend));

== matlab function indy7_dualArm/Subsystem/MATLAB Function1 ==
  data: R_start input; R_t output; xi_t input; omega_t output; omegadot_t output; xidot_t input; xiddot_t input
function [R_t,omega_t,omegadot_t] = ExpCoordinateToSO3(R_start,xi_t,xidot_t,xiddot_t)
R_t = eye(3);
omega_t = zeros(3,1);
omegadot_t = zeros(3,1);


R_t = R_start*MatrixExp3(VecToso3(xi_t));
omega_t = dexp3(-xi_t)*xidot_t;
omegadot_t = dexp3(-xi_t)*xiddot_t+ ddexp3(-xi_t,-xidot_t)*xidot_t;

== matlab function indy7_dualArm/Subsystem/TransToRp ==
  data: T input; R output; p output
function [R,p] = TransToRp(T)

[R,p] = TransToRp(T);

== matlab function indy7_dualArm/Subsystem/TransToRp1 ==
  data: T input; R output; p output
function [R,p] = TransToRp(T)

[R,p] = TransToRp(T);

== matlab function indy7_dualArm/DualArmTaskSpaceController/SPDControllerWithQP_Left1 ==
  data: M input; cvec input; q input size=[12,1]; qddot output size=[6,1]; qdot input size=[12,1]; Tdes input size=[4,4]; Vdes input size=[6,1]; Vdotdes input size=[6,1]; T input size=[4,4]; V input size=[6,1]; J input size=[6,6]; Jdot input size=[6,6]; qinit input size=[6,1]; qdot_max input size=[6,1]; qdot_min input size=[6,1]; q_max input size=[6,1]; q_min input size=[6,1]; TaskKp input size=[1,6]; TaskKv input size=[1,6]; dt input; a input; b0 input
function qddot = SPDImplicitEuler(M,cvec,q,qdot,Tdes,Vdes,Vdotdes,T,V,J,Jdot,qinit,qdot_max,qdot_min,q_max,q_min,TaskKp,TaskKv,dt,a,b0)
    % Tdes(2,4) = Tdes(2,4)+0.3*sin(2*pi*t/5);
    M = M(7:end,7:end);
    qdot  = qdot(7:end);
    q = q(7:end);
    cvec = cvec(7:end);

    % % Tdes(3,4) = Tdes(3,4)+0.5*sin(2*pi*t/5);

    TaskKp = diag(TaskKp);
    TaskKv = diag(TaskKv);


    Ttilde = TransInv(T)*Tdes;
    lambda  = log6(Ttilde);
    Vtilde = Vdes-Adjoint(TransInv(Ttilde))*V;
    dlambda = dexp6(-lambda)*Vtilde;
    AdInvT = Adjoint(TransInv(Ttilde));
    D = dlog6(-lambda)*Vdotdes-dlog6(-lambda)*AdInvT*Jdot*qdot+dlog6(-lambda)*ad(Vtilde)*Vdes-dlog6(-lambda)*ddexp6(-lambda,-dlambda)*dlambda;
    % qddot = (M+JT*TaskKv*dt*dlog6(-lambda)*AdInvT*J)\(JT*TaskKp*(lambda)+JT*TaskKp*dt*dlambda+JT*TaskKv*dlambda+(eye(7)-pinv(J)*J)*(Kinit*(qinit-q)+Dinit*(-qdot))-B*qdot);
    
    
      
    Jlambda = -dlog6(lambda)*J;
    Vtilde = Adjoint(TransInv(Ttilde))*Vdes-V;
    lambdadot = dlog6(lambda)*Vtilde;
    lambda_next = lambda+lambdadot*dt;
    B = b0 * exp(-det(J)*det(J)/ a / a) * eye(length(q));

    JlambdaT = Jlambda';
    Gamma = dlog6(lambda_next)*Adjoint(exp6(-lambda_next))*(Vdes+dt*Vdotdes)-dlog6(lambda_next)*V-dlog6(lambda_next)*dt*Jdot*qdot;
    qddot = (M+JlambdaT*TaskKv*dt*Jlambda)\(JlambdaT*(-TaskKp*lambda_next-TaskKv*Gamma)-cvec-B*qdot);


    % Js_prime= JacobianSpace(Slist6,q(2:end));
    % Jsdot_prime= dJacobianSpace(Js_prime,qdot(2:end));
    % Tbase_tcp =FKinSpace(M_tcp,Slist6,q(2:end));
    % p = Tbase_tcp(1:3,4);
    % pdot = Js_prime(1:3,:)*qdot(2:end);
    % 
    % 
    % p_max = 2.5;
    % lambda = 0.1;
    % 
    H = eye(6);
    % H = H+lambda*eye(6);

    f = -2*qddot;
    % f = f-lambda*qddot_prev;
    % Ao = Js_prime(1,:)*[zeros(6,1) eye(6)];

    Au = eye(6);
    bu = 10*[qdot_max-qdot];
    bl = -10*[qdot-qdot_min];
    alpha1 = 1;
    alpha3 = 10;
    beta1 = 10;
    beta3 = 100;
    Aq =eye(6);
    bqu = [-(alpha1+alpha3)*qdot+(alpha1*alpha3)*(q_max-q)];
    bql = [-(alpha1+alpha3)*qdot-(alpha1*alpha3)*(q-q_min)];
    % bou = [-(beta1+beta3)*pdot(1)+(beta1*beta3)*(p_max-p(1))-Jsdot_prime(1,:)*qdot(2:end)];

    x0 = qddot;

    A = [Au;-Au;Aq;-Aq];
    b = [bu;-bl;bqu;-bql];
    % A = [Au;-Au;Aq;-Aq];
    % b = [bu;-bl;bqu;-bql];
    options = optimoptions('quadprog', ...
                           'Algorithm','active-set', ...
                           'Display','off');

    % 4) quadprog 호출
    [x, fval, exitflag, output, lambda] = quadprog( ...
        H, f, A, b, [], [], [], [], x0, options);
    if(exitflag>0)
        qddot =x;
    else

    end

== matlab function indy7_dualArm/MATLAB Function ==
  data: Tl input; Tlr output; Tr input; Trl output
function [Tlr,Trl] = fcn(Tl,Tr)

Tlr= TransInv(Tl)*Tr;
Trl=TransInv(Tlr);

== matlab function indy7_dualArm/Subsystem1/GetT,V,Vdot ==
  data: p_t input; T_t output; pdot_t input; pddot_t input; R_t input; omega_t input; omegadot_t input; V_t output; Vdot_t output
function [T_t,V_t,Vdot_t] = getTVVdot(p_t,pdot_t,pddot_t,R_t,omega_t,omegadot_t)

T_t = RpToTrans(R_t,p_t);
V_t = [R_t'*pdot_t;omega_t];
Rdot_t = (R_t*VecToso3(omega_t))';
Vdot_t = [Rdot_t'*pdot_t+R_t'*pddot_t;omegadot_t];

== matlab function indy7_dualArm/Subsystem1/MATLAB Function ==
  data: Rstart input; xi_start output; Rend input; xi_end output
function [xi_start,xi_end] = fcn(Rstart,Rend)

xi_start = zeros(3,1);
xi_end = zeros(3,1);

xi_end = so3ToVec(MatrixLog3((Rstart)'*Rend));

== matlab function indy7_dualArm/Subsystem1/MATLAB Function1 ==
  data: R_start input; R_t output; xi_t input; omega_t output; omegadot_t output; xidot_t input; xiddot_t input
function [R_t,omega_t,omegadot_t] = ExpCoordinateToSO3(R_start,xi_t,xidot_t,xiddot_t)
R_t = eye(3);
omega_t = zeros(3,1);
omegadot_t = zeros(3,1);


R_t = R_start*MatrixExp3(VecToso3(xi_t));
omega_t = dexp3(-xi_t)*xidot_t;
omegadot_t = dexp3(-xi_t)*xiddot_t+ ddexp3(-xi_t,-xidot_t)*xidot_t;

== matlab function indy7_dualArm/Subsystem1/TransToRp ==
  data: T input; R output; p output
function [R,p] = TransToRp(T)

[R,p] = TransToRp(T);

== matlab function indy7_dualArm/Subsystem1/TransToRp1 ==
  data: T input; R output; p output
function [R,p] = TransToRp(T)

[R,p] = TransToRp(T);

== matlab function indy7_dualArm/SPDController/ForwardKinematics(510) ==
  data: q input; T output; qdot input; V output; Vdot output; J output; Jdot output; M input; Blist input
function [T,V,Vdot,J,Jdot] = ForwardKinematics(q,qdot,M,Blist)
T = eye(4);
V = zeros(6,1);
Vdot=zeros(6,1);
J = zeros(6,7);
Jdot = zeros(6,7);

T = FKinBody(M,Blist,q);    
J = JacobianBody(Blist,q);
V = J*qdot;
Jdot = dJacobianBody(J,qdot);

== matlab function indy7_dualArm/SPDController/ImpedaceModel ==
  data: x_state input size=[12,1]; T_des_prime output size=[4,4]; T_des input size=[4,4]; V_des input size=[6,1]; Vdot_des input size=[6,1]; Fdes input size=[6,1]; V_des_prime output size=[6,1]; Vdot_des_prime output size=[6,1]; Fext input size=[6,1]; dt input; x_state output; Avec input size=[6,1]; Dvec input size=[6,1]; Kvec input size=[6,1]; lambda_max input size=[6,1]; lambda_min input size=[6,1]
function [T_des_prime,V_des_prime,Vdot_des_prime,x_state] =ImpedanceModel(x_state,T_des,V_des,Vdot_des,Fdes,Fext,dt,Avec,Dvec,Kvec,lambda_max,lambda_min)
    
    %% Initialize
    T_des_prime = eye(4);
    V_des_prime = zeros(6,1);
    Vdot_des_prime = zeros(6,1);
    Ferr = Fext - Fdes;
    [t_,x_dot] = ode45(@(t_,x_dot) SingleBodyDynamics(t_,x_state,Ferr,Avec,Dvec,Kvec,lambda_max,lambda_min),[0, dt] , x_state ); 
    p = x_state(1:3);    
    xi = x_state(4:6);
    pdot = x_state(7:9);
    xidot = x_state(10:12);
    x_state = x_dot(end,:)';
    pddot=(diag(Avec(1:3)))\(Ferr(1:3)-diag(Dvec(1:3))*pdot - diag(Kvec(1:3))*p);
    xiddot=(diag(Avec(4:6)))\(Ferr(4:6)-diag(Dvec(4:6))*xidot - diag(Kvec(4:6))*p);
  
    
    eta = dlog3(xi)*p;
    etadot = ddlog3(xi,xidot)*p+dlog3(xi)*pdot;
    etaddot = dddexpInvSo3(xi,xidot,xiddot)*p+2*ddlog3(xi,xidot)*pdot+dlog3(xi)*pddot;
    
    lambda = [eta;xi];
    lambdadot = [etadot;xidot];
    lambdaddot = [etaddot;xiddot];
    T_tilde_prime = exp6(lambda);
    V_tilde_prime = dexp6(lambda)*lambdadot;
    Vdot_tilde_prime = ddexp6(lambda,lambdadot)*lambdadot+dexp6(lambda)*lambdaddot;
    T_des_prime = T_des*T_tilde_prime;
    V_des_prime = Adjoint(TransInv(T_tilde_prime))*(V_tilde_prime+V_des);
    Vdot_des_prime=Adjoint(TransInv(T_tilde_prime))*(Vdot_tilde_prime-ad(V_tilde_prime)*V_des_prime+Vdot_des);
end

function xdot = SingleBodyDynamics(t, x, F,Avec,Dvec,Kvec,lambda_max,lambda_min)

    lambda    = x(1:6);
    lambdadot = x(7:12);
    A = diag(Avec);
    D = diag(Dvec);
    K = diag(Kvec);
    
    Spring = (K*lambda);
    
    F(4:6) = dexp3(-lambda(4:6))'*F(4:6);

    lambdaddot = A \ (F - D*lambdadot - Spring);
    H = eye(6);
    f = -2*lambdaddot;
    Au = eye(6);
    alpha1 = 1;
    alpha3 = 10;
    bl = -(alpha1 + alpha3)*lambdadot-(alpha1*alpha3)*(lambda-lambda_min);
    bu = -(alpha1 + alpha3)*lambdadot+(alpha1*alpha3)*(lambda_max-lambda);

    x0 = lambdaddot;
    
    A = [Au;-Au;];
    b = [bu;-bl;];
    options = optimoptions('quadprog', ...
                           'Algorithm','active-set', ...
                           'Display','off');

    % 4) quadprog 호출
    [x, fval, exitflag, output, lambda] = quadprog( ...
        H, f, A, b, [], [], [], [], x0, options);
    if exitflag>0
        lambdaddot =x;
    end
    


    xdot = [lambdadot;
          lambdaddot];
end

== matlab function indy7_dualArm/SPDController/SPDControllerWithQP ==
  data: M input; cvec input; q input size=[7,1]; qddot output size=[7,1]; qdot input size=[7,1]; Tdes input size=[4,4]; Vdes input size=[6,1]; Vdotdes input size=[6,1]; T input size=[4,4]; V input size=[6,1]; J input size=[6,7]; Jdot input size=[6,7]; qinit input size=[7,1]; qdot_max input size=[7,1]; qdot_min input size=[7,1]; q_max input size=[7,1]; q_min input size=[7,1]; Kinit input size=[7,1]; Dinit input size=[7,1]; TaskKp input size=[1,6]; TaskKv input size=[1,6]; dt input; a input; b0 input; Slist6 input; M_tcp input; qddot_prev input
function qddot = SPDImplicitEuler(M,cvec,q,qdot,Tdes,Vdes,Vdotdes,T,V,J,Jdot,qinit,qdot_max,qdot_min,q_max,q_min,Kinit,Dinit,TaskKp,TaskKv,dt,a,b0,Slist6, M_tcp,qddot_prev)
    % Tdes(2,4) = Tdes(2,4)+0.3*sin(2*pi*t/5);
    % % Tdes(3,4) = Tdes(3,4)+0.5*sin(2*pi*t/5);
    % Kinit = zeros(7,1);
    % Dinit = zeros(7,1);
    Kinit = diag(Kinit);
    Dinit = diag(Dinit);
    TaskKp = diag(TaskKp);
    TaskKv = diag(TaskKv);


    Ttilde = TransInv(T)*Tdes;
    lambda  = log6(Ttilde);
    Vtilde = Vdes-Adjoint(TransInv(Ttilde))*V;
    dlambda = dexp6(-lambda)*Vtilde;
    AdInvT = Adjoint(TransInv(Ttilde));
    D = dlog6(-lambda)*Vdotdes-dlog6(-lambda)*AdInvT*Jdot*qdot+dlog6(-lambda)*ad(Vtilde)*Vdes-dlog6(-lambda)*ddexp6(-lambda,-dlambda)*dlambda;
    B = b0*exp(-det(J(1:6,1:6))*det(J(1:6,1:6))/a/a)*eye(6);
    % qddot = (M+JT*TaskKv*dt*dlog6(-lambda)*AdInvT*J)\(JT*TaskKp*(lambda)+JT*TaskKp*dt*dlambda+JT*TaskKv*dlambda+(eye(7)-pinv(J)*J)*(Kinit*(qinit-q)+Dinit*(-qdot))-B*qdot);
    
    
      
    Jlambda = -dlog6(lambda)*J;
    Vtilde = Adjoint(TransInv(Ttilde))*Vdes-V;
    lambdadot = dlog6(lambda)*Vtilde;
    lambda_next = lambda+lambdadot*dt;
    B = b0 * exp(-det(J(1:end,2:end))*det(J(1:end,2:end))/ a / a) * eye(length(q));

    JlambdaT = Jlambda';
    Gamma = dlog6(lambda_next)*Adjoint(exp6(-lambda_next))*(Vdes+dt*Vdotdes)-dlog6(lambda_next)*V-dlog6(lambda_next)*dt*Jdot*qdot;
    qddot = (M+JlambdaT*TaskKv*dt*Jlambda)\(JlambdaT*(-TaskKp*lambda_next-TaskKv*Gamma)+(eye(7)-pinv(J)*J)*((Kinit)*(qinit-q)+(Dinit)*(-qdot))-cvec-B*qdot);


    Js_prime= JacobianSpace(Slist6,q(2:end));
    Jsdot_prime= dJacobianSpace(Js_prime,qdot(2:end));
    Tbase_tcp =FKinSpace(M_tcp,Slist6,q(2:end));
    p = Tbase_tcp(1:3,4);
    pdot = Js_prime(1:3,:)*qdot(2:end);
    

    p_max = 2.5;
    lambda = 0.1;

    H = eye(7);
    H = H+lambda*eye(7);

    f = -2*qddot;
    f = f-lambda*qddot_prev;
    Ao = Js_prime(1,:)*[zeros(6,1) eye(6)];

    Au = eye(7);
    bu = 10*[qdot_max-qdot];
    bl = -10*[qdot-qdot_min];
    alpha1 = 1;
    alpha3 = 10;
    beta1 = 10;
    beta3 = 100;
    Aq =eye(7);
    bqu = [-(alpha1+alpha3)*qdot+(alpha1*alpha3)*(q_max-q)];
    bql = [-(alpha1+alpha3)*qdot-(alpha1*alpha3)*(q-q_min)];
    bou = [-(beta1+beta3)*pdot(1)+(beta1*beta3)*(p_max-p(1))-Jsdot_prime(1,:)*qdot(2:end)];

    x0 = qddot;
    
    A = [Au;-Au;Aq;-Aq];
    b = [bu;-bl;bqu;-bql];
    % A = [Au;-Au;Aq;-Aq];
    % b = [bu;-bl;bqu;-bql];
    options = optimoptions('quadprog', ...
                           'Algorithm','active-set', ...
                           'Display','off');

    % 4) quadprog 호출
    [x, fval, exitflag, output, lambda] = quadprog( ...
        H, f, A, b, [], [], [], [], x0, options);
    if(exitflag>0)
        qddot =x;
    else
        
    end
